simulink model "LogicalArchitecture"  (R2020b)
settings: Solver=VariableStepAuto  StartTime=0.0  StopTime=10.0  RelTol=1e-3
settings Model: DataDictionary=SignalInterfacesDD.sldd  OrderedModelArguments=off  Creator=jantonio  LastModifiedBy=jantonio

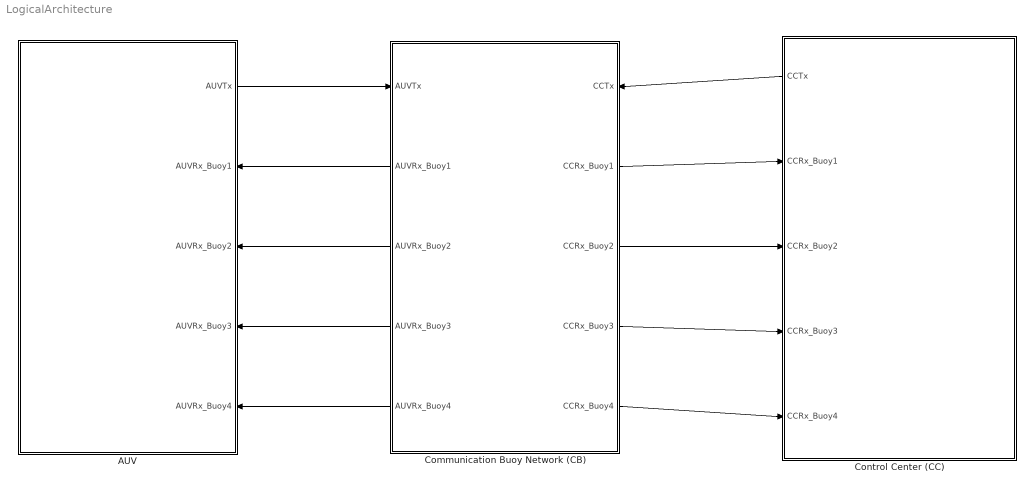
== system LogicalArchitecture ==
  AUV : Subsystem
      settings: PortSchema="{\"entries\":[{\"content\":{\"headerSize\":26,\"margin\":15,\"minimumSpacing\":25,\"sides\":[{\"content\":{\"connectorIds\":[]},\"type\":\"ConnectorPlacement.EquallySpacedRectSide\",\"uuid\":\"7765e1d4-0dc4-4e3a-8ace-6707e97be0d4\"},{\"content\":{\"connectorIds\":[\"Out1\",\"In1\",\"In2\",\"In3\",\"In4\"],\"side\":\"RIGHT\"},\"type\":\"ConnectorPlacement.EquallySpacedRectSide\",\"uuid\":\"17453679-37e1-41d9-ae4d-157eecb5c7d5\"},{\"content\":{\"connectorIds\":[],\"side\":\"TOP\"},\"type\":\"ConnectorPlacement.EquallySpacedRectSide\",\"uuid\":\"00031b71-5a14-4188-ab65-fea9bc3c8fe0\"},{\"content\":{\"connectorIds\":[],\"side\":\"HIDDEN\"},\"type\":\"ConnectorPlacement.EquallySpacedRectSide\",\"uuid\":\"5a9649b7-70c5-4a2b-8171-d74ca0553427\"}]},\"type\":\"ConnectorPlacement.EquallySpacedConnector\",\"uuid\":\"792023c5-1206-4f5a-b9db-8c0c10ca5715\"}],\"packageUris\":[\"http://schema.mathworks.com/mf0/Connector/R2020b\"],\"version\":\"1.0\"}"
  Communication Buoy Network (CB) : Subsystem
      settings: PortSchema="{\"entries\":[{\"content\":{\"headerSize\":26,\"margin\":15,\"minimumSpacing\":25,\"sides\":[{\"content\":{\"connectorIds\":[\"In1\",\"Out5\",\"Out8\",\"Out7\",\"Out6\"]},\"type\":\"ConnectorPlacement.EquallySpacedRectSide\",\"uuid\":\"7765e1d4-0dc4-4e3a-8ace-6707e97be0d4\"},{\"content\":{\"connectorIds\":[\"In2\",\"Out1\",\"Out2\",\"Out3\",\"Out4\"],\"side\":\"RIGHT\"},\"type\":\"ConnectorPlacement.EquallySpacedRectSide\",\"uuid\":\"17453679-37e1-41d9-ae4d-157eecb5c7d5\"},{\"content\":{\"connectorIds\":[],\"side\":\"TOP\"},\"type\":\"ConnectorPlacement.EquallySpacedRectSide\",\"uuid\":\"00031b71-5a14-4188-ab65-fea9bc3c8fe0\"},{\"content\":{\"connectorIds\":[],\"side\":\"HIDDEN\"},\"type\":\"ConnectorPlacement.EquallySpacedRectSide\",\"uuid\":\"5a9649b7-70c5-4a2b-8171-d74ca0553427\"}]},\"type\":\"ConnectorPlacement.EquallySpacedConnector\",\"uuid\":\"792023c5-1206-4f5a-b9db-8c0c10ca5715\"}],\"packageUris\":[\"http://schema.mathworks.com/mf0/Connector/R2020b\"],\"version\":\"1.0\"}"
  Control Center (CC) : Subsystem
      settings: PortSchema="{\"entries\":[{\"content\":{\"headerSize\":26,\"margin\":15,\"minimumSpacing\":25,\"sides\":[{\"content\":{\"connectorIds\":[\"Out1\",\"In1\",\"In2\",\"In3\",\"In4\"]},\"type\":\"ConnectorPlacement.EquallySpacedRectSide\",\"uuid\":\"5928ce2f-b7da-4eaf-83b8-f1dfd8275719\"},{\"content\":{\"connectorIds\":[],\"side\":\"RIGHT\"},\"type\":\"ConnectorPlacement.EquallySpacedRectSide\",\"uuid\":\"1e52cfd1-9d99-4f69-bb2a-b495e37ce87e\"},{\"content\":{\"connectorIds\":[],\"side\":\"TOP\"},\"type\":\"ConnectorPlacement.EquallySpacedRectSide\",\"uuid\":\"b4ddd4ca-36f1-4266-858a-a649bf629535\"},{\"content\":{\"connectorIds\":[],\"side\":\"HIDDEN\"},\"type\":\"ConnectorPlacement.EquallySpacedRectSide\",\"uuid\":\"84c51e85-8df3-4dbb-bd65-3b1aecd54e94\"}]},\"type\":\"ConnectorPlacement.EquallySpacedConnector\",\"uuid\":\"e0d55cd3-5fe9-4d4e-95d9-79589f5b6259\"}],\"packageUris\":[\"http://schema.mathworks.com/mf0/Connector/R2020b\"],\"version\":\"1.0\"}"
  wires:
  AUV/1(AUVTx) -> Communication Buoy Network (CB)/1(AUVTx)
  Control Center (CC)/1(CCTx) -> Communication Buoy Network (CB)/2(CCTx)
  Communication Buoy Network (CB)/5(AUVRx_Buoy1) -> AUV/1(AUVRx_Buoy1)
  Communication Buoy Network (CB)/8(AUVRx_Buoy2) -> AUV/2(AUVRx_Buoy2)
  Communication Buoy Network (CB)/7(AUVRx_Buoy3) -> AUV/3(AUVRx_Buoy3)
  Communication Buoy Network (CB)/6(AUVRx_Buoy4) -> AUV/4(AUVRx_Buoy4)
  Communication Buoy Network (CB)/1(CCRx_Buoy1) -> Control Center (CC)/1(CCRx_Buoy1)
  Communication Buoy Network (CB)/2(CCRx_Buoy2) -> Control Center (CC)/2(CCRx_Buoy2)
  Communication Buoy Network (CB)/3(CCRx_Buoy3) -> Control Center (CC)/3(CCRx_Buoy3)
  Communication Buoy Network (CB)/4(CCRx_Buoy4) -> Control Center (CC)/4(CCRx_Buoy4)

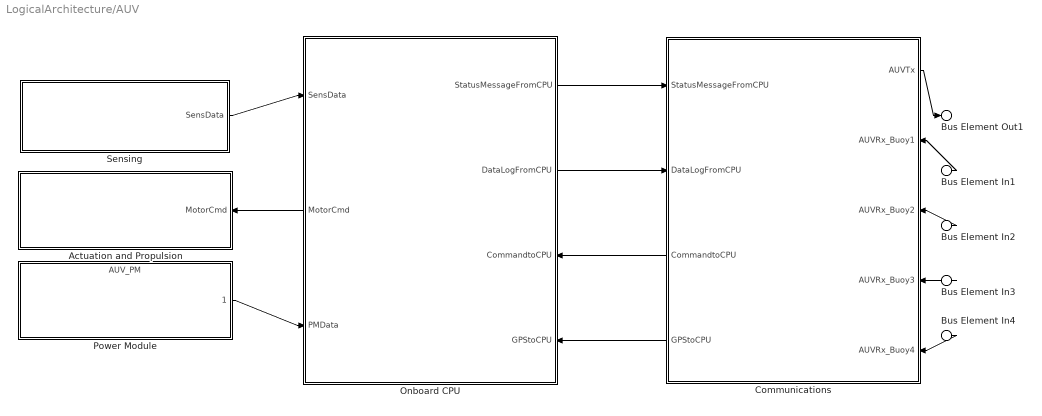
== system LogicalArchitecture/AUV ==
  Bus Element In1 : Inport  PortName=AUVRx_Buoy1
  Bus Element In2 : Inport  Port=2  PortName=AUVRx_Buoy2
  Bus Element In3 : Inport  Port=3  PortName=AUVRx_Buoy3
  Bus Element In4 : Inport  Port=4  PortName=AUVRx_Buoy4
  Actuation and Propulsion : Subsystem
      settings: PortSchema="{\"entries\":[{\"content\":{\"headerSize\":26,\"margin\":15,\"minimumSpacing\":25,\"sides\":[{\"content\":{\"connectorIds\":[]},\"type\":\"ConnectorPlacement.EquallySpacedRectSide\",\"uuid\":\"7765e1d4-0dc4-4e3a-8ace-6707e97be0d4\"},{\"content\":{\"connectorIds\":[\"In1\"],\"side\":\"RIGHT\"},\"type\":\"ConnectorPlacement.EquallySpacedRectSide\",\"uuid\":\"17453679-37e1-41d9-ae4d-157eecb5c7d5\"},{\"content\":{\"connectorIds\":[],\"side\":\"TOP\"},\"type\":\"ConnectorPlacement.EquallySpacedRectSide\",\"uuid\":\"00031b71-5a14-4188-ab65-fea9bc3c8fe0\"},{\"content\":{\"connectorIds\":[],\"side\":\"HIDDEN\"},\"type\":\"ConnectorPlacement.EquallySpacedRectSide\",\"uuid\":\"5a9649b7-70c5-4a2b-8171-d74ca0553427\"}]},\"type\":\"ConnectorPlacement.EquallySpacedConnector\",\"uuid\":\"792023c5-1206-4f5a-b9db-8c0c10ca5715\"}],\"packageUris\":[\"http://schema.mathworks.com/mf0/Connector/R2020b\"],\"version\":\"1.0\"}"
  Communications : Subsystem
      settings: PortSchema="{\"entries\":[{\"content\":{\"headerSize\":26,\"margin\":15,\"minimumSpacing\":25,\"sides\":[{\"content\":{\"connectorIds\":[\"In1\",\"In2\",\"Out2\",\"Out3\"]},\"type\":\"ConnectorPlacement.EquallySpacedRectSide\",\"uuid\":\"5928ce2f-b7da-4eaf-83b8-f1dfd8275719\"},{\"content\":{\"connectorIds\":[\"Out1\",\"In3\",\"In6\",\"In5\",\"In4\"],\"side\":\"RIGHT\"},\"type\":\"ConnectorPlacement.EquallySpacedRectSide\",\"uuid\":\"1e52cfd1-9d99-4f69-bb2a-b495e37ce87e\"},{\"content\":{\"connectorIds\":[],\"side\":\"TOP\"},\"type\":\"ConnectorPlacement.EquallySpacedRectSide\",\"uuid\":\"b4ddd4ca-36f1-4266-858a-a649bf629535\"},{\"content\":{\"connectorIds\":[],\"side\":\"HIDDEN\"},\"type\":\"ConnectorPlacement.EquallySpacedRectSide\",\"uuid\":\"84c51e85-8df3-4dbb-bd65-3b1aecd54e94\"}]},\"type\":\"ConnectorPlacement.EquallySpacedConnector\",\"uuid\":\"e0d55cd3-5fe9-4d4e-95d9-79589f5b6259\"}],\"packageUris\":[\"http://schema.mathworks.com/mf0/Connector/R2020b\"],\"version\":\"1.0\"}"
  Onboard CPU : Subsystem
      settings: PortSchema="{\"entries\":[{\"content\":{\"headerSize\":26,\"margin\":15,\"minimumSpacing\":25,\"sides\":[{\"content\":{\"connectorIds\":[\"In3\",\"Out1\",\"In4\"]},\"type\":\"ConnectorPlacement.EquallySpacedRectSide\",\"uuid\":\"7765e1d4-0dc4-4e3a-8ace-6707e97be0d4\"},{\"content\":{\"connectorIds\":[\"Out3\",\"Out2\",\"In1\",\"In2\"],\"side\":\"RIGHT\"},\"type\":\"ConnectorPlacement.EquallySpacedRectSide\",\"uuid\":\"17453679-37e1-41d9-ae4d-157eecb5c7d5\"},{\"content\":{\"connectorIds\":[],\"side\":\"TOP\"},\"type\":\"ConnectorPlacement.EquallySpacedRectSide\",\"uuid\":\"00031b71-5a14-4188-ab65-fea9bc3c8fe0\"},{\"content\":{\"connectorIds\":[],\"side\":\"HIDDEN\"},\"type\":\"ConnectorPlacement.EquallySpacedRectSide\",\"uuid\":\"5a9649b7-70c5-4a2b-8171-d74ca0553427\"}]},\"type\":\"ConnectorPlacement.EquallySpacedConnector\",\"uuid\":\"792023c5-1206-4f5a-b9db-8c0c10ca5715\"}],\"packageUris\":[\"http://schema.mathworks.com/mf0/Connector/R2020b\"],\"version\":\"1.0\"}"
  Power Module : ModelReference  ModelNameDialog=AUV_PM  SimulationMode=Normal  ModelReferenceVersion=1.7
      settings: PortSchema="{\"entries\":[{\"content\":{\"headerSize\":38,\"margin\":15,\"minimumSpacing\":25,\"sides\":[{\"content\":{\"connectorIds\":[]},\"type\":\"ConnectorPlacement.EquallySpacedRectSide\",\"uuid\":\"7765e1d4-0dc4-4e3a-8ace-6707e97be0d4\"},{\"content\":{\"connectorIds\":[\"Out1\"],\"side\":\"RIGHT\"},\"type\":\"ConnectorPlacement.EquallySpacedRectSide\",\"uuid\":\"17453679-37e1-41d9-ae4d-157eecb5c7d5\"},{\"content\":{\"connectorIds\":[],\"side\":\"TOP\"},\"type\":\"ConnectorPlacement.EquallySpacedRectSide\",\"uuid\":\"00031b71-5a14-4188-ab65-fea9bc3c8fe0\"},{\"content\":{\"connectorIds\":[],\"side\":\"HIDDEN\"},\"type\":\"ConnectorPlacement.EquallySpacedRectSide\",\"uuid\":\"5a9649b7-70c5-4a2b-8171-d74ca0553427\"}]},\"type\":\"ConnectorPlacement.EquallySpacedConnector\",\"uuid\":\"792023c5-1206-4f5a-b9db-8c0c10ca5715\"}],\"packageUris\":[\"http://schema.mathworks.com/mf0/Connector/R2020b\"],\"version\":\"1.0\"}"
  Sensing : Subsystem
      settings: PortSchema="{\"entries\":[{\"content\":{\"headerSize\":26,\"margin\":15,\"minimumSpacing\":25,\"sides\":[{\"content\":{\"connectorIds\":[]},\"type\":\"ConnectorPlacement.EquallySpacedRectSide\",\"uuid\":\"7765e1d4-0dc4-4e3a-8ace-6707e97be0d4\"},{\"content\":{\"connectorIds\":[\"Out1\"],\"side\":\"RIGHT\"},\"type\":\"ConnectorPlacement.EquallySpacedRectSide\",\"uuid\":\"17453679-37e1-41d9-ae4d-157eecb5c7d5\"},{\"content\":{\"connectorIds\":[],\"side\":\"TOP\"},\"type\":\"ConnectorPlacement.EquallySpacedRectSide\",\"uuid\":\"00031b71-5a14-4188-ab65-fea9bc3c8fe0\"},{\"content\":{\"connectorIds\":[],\"side\":\"HIDDEN\"},\"type\":\"ConnectorPlacement.EquallySpacedRectSide\",\"uuid\":\"5a9649b7-70c5-4a2b-8171-d74ca0553427\"}]},\"type\":\"ConnectorPlacement.EquallySpacedConnector\",\"uuid\":\"792023c5-1206-4f5a-b9db-8c0c10ca5715\"}],\"packageUris\":[\"http://schema.mathworks.com/mf0/Connector/R2020b\"],\"version\":\"1.0\"}"
  Bus Element Out1 : Outport  PortName=AUVTx
  wires:
  Power Module/1 -> Onboard CPU/4(PMData)
  Sensing/1(SensData) -> Onboard CPU/3(SensData)
  Onboard CPU/1(MotorCmd) -> Actuation and Propulsion/1(MotorCmd)
  Bus Element In1/1 -> Communications/3(AUVRx_Buoy1)
  Bus Element In2/1 -> Communications/6(AUVRx_Buoy2)
  Bus Element In3/1 -> Communications/5(AUVRx_Buoy3)
  Bus Element In4/1 -> Communications/4(AUVRx_Buoy4)
  Onboard CPU/2(DataLogFromCPU) -> Communications/2(DataLogFromCPU)
  Onboard CPU/3(StatusMessageFromCPU) -> Communications/1(StatusMessageFromCPU)
  Communications/1(AUVTx) -> Bus Element Out1/1
  Communications/2(CommandtoCPU) -> Onboard CPU/1(CommandtoCPU)
  Communications/3(GPStoCPU) -> Onboard CPU/2(GPStoCPU)

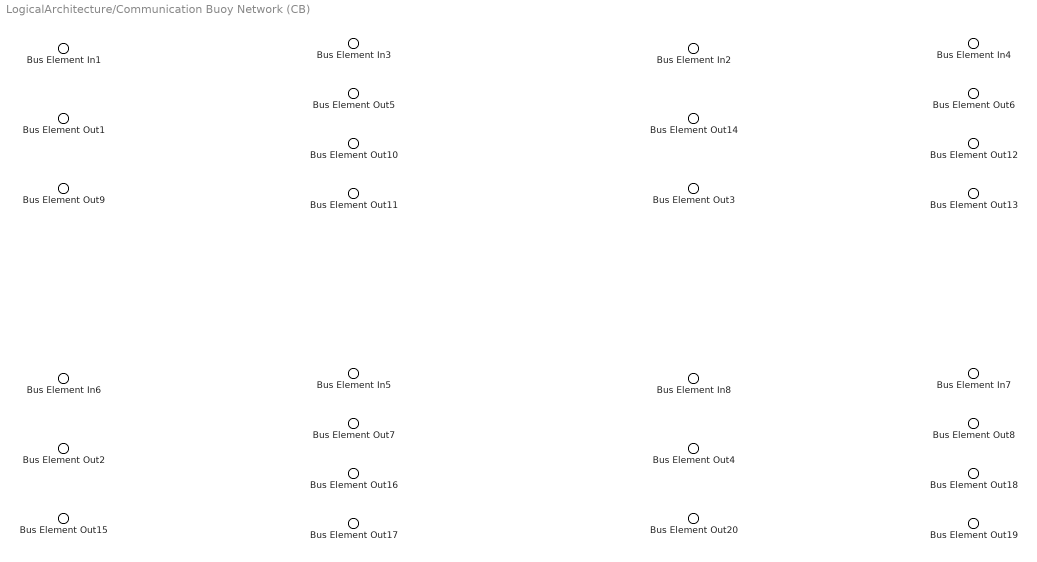
== system LogicalArchitecture/Communication Buoy Network (CB) ==
  Bus Element In{1..2,6,8} (4 alike) : Inport  PortName=AUVTx
  Bus Element In{3..5,7} (4 alike) : Inport  Port=2  PortName=CCTx
  Bus Element Out5 : Outport  PortName=CCRx_Buoy1  Element=StatusMessage
  Bus Element Out10 : Outport  PortName=CCRx_Buoy1  Element=GPS
  Bus Element Out11 : Outport  PortName=CCRx_Buoy1  Element=PowerStatus
  Bus Element Out6 : Outport  Port=2  PortName=CCRx_Buoy2  Element=StatusMessage
  Bus Element Out12 : Outport  Port=2  PortName=CCRx_Buoy2  Element=GPS
  Bus Element Out13 : Outport  Port=2  PortName=CCRx_Buoy2  Element=PowerStatus
  Bus Element Out7 : Outport  Port=3  PortName=CCRx_Buoy3  Element=StatusMessage
  Bus Element Out16 : Outport  Port=3  PortName=CCRx_Buoy3  Element=GPS
  Bus Element Out17 : Outport  Port=3  PortName=CCRx_Buoy3  Element=PowerStatus
  Bus Element Out8 : Outport  Port=4  PortName=CCRx_Buoy4  Element=StatusMessage
  Bus Element Out18 : Outport  Port=4  PortName=CCRx_Buoy4  Element=GPS
  Bus Element Out19 : Outport  Port=4  PortName=CCRx_Buoy4  Element=PowerStatus
  Bus Element Out1 : Outport  Port=5  PortName=AUVRx_Buoy1  Element=GPS
  Bus Element Out9 : Outport  Port=5  PortName=AUVRx_Buoy1  Element=Command
  Bus Element Out4 : Outport  Port=6  PortName=AUVRx_Buoy4  Element=GPS
  Bus Element Out20 : Outport  Port=6  PortName=AUVRx_Buoy4  Element=Command
  Bus Element Out2 : Outport  Port=7  PortName=AUVRx_Buoy3  Element=GPS
  Bus Element Out15 : Outport  Port=7  PortName=AUVRx_Buoy3  Element=Command
  Bus Element Out14 : Outport  Port=8  PortName=AUVRx_Buoy2  Element=GPS
  Bus Element Out3 : Outport  Port=8  PortName=AUVRx_Buoy2  Element=Command

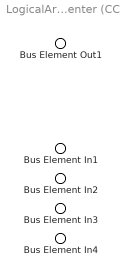
== system LogicalArchitecture/Control Center (CC) ==
  Bus Element In1 : Inport  PortName=CCRx_Buoy1
  Bus Element In2 : Inport  Port=2  PortName=CCRx_Buoy2
  Bus Element In3 : Inport  Port=3  PortName=CCRx_Buoy3
  Bus Element In4 : Inport  Port=4  PortName=CCRx_Buoy4
  Bus Element Out1 : Outport  PortName=CCTx  Element=Command

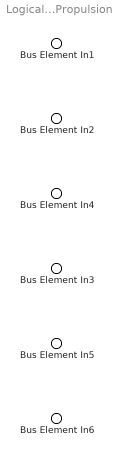
== system LogicalArchitecture/AUV/Actuation and Propulsion ==
  Bus Element In1 : Inport  PortName=MotorCmd  Element=HT1
  Bus Element In2 : Inport  PortName=MotorCmd  Element=HT2
  Bus Element In4 : Inport  PortName=MotorCmd  Element=VT1
  Bus Element In3 : Inport  PortName=MotorCmd  Element=VT2
  Bus Element In5 : Inport  PortName=MotorCmd  Element=MT1
  Bus Element In6 : Inport  PortName=MotorCmd  Element=MT2

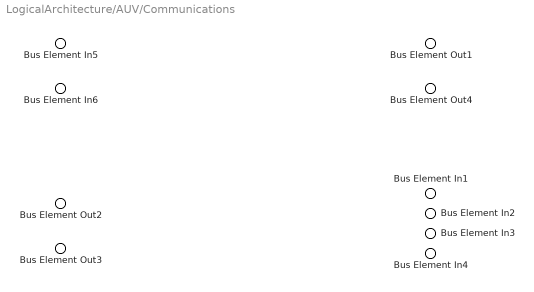
== system LogicalArchitecture/AUV/Communications ==
  Bus Element In5 : Inport  PortName=StatusMessageFromCPU
  Bus Element In6 : Inport  Port=2  PortName=DataLogFromCPU
  Bus Element In1 : Inport  Port=3  PortName=AUVRx_Buoy1
  Bus Element In4 : Inport  Port=4  PortName=AUVRx_Buoy4
  Bus Element In3 : Inport  Port=5  PortName=AUVRx_Buoy3
  Bus Element In2 : Inport  Port=6  PortName=AUVRx_Buoy2
  Bus Element Out1 : Outport  PortName=AUVTx  Element=StatusMessage
  Bus Element Out4 : Outport  PortName=AUVTx  Element=DataLog
  Bus Element Out2 : Outport  Port=2  PortName=CommandtoCPU
  Bus Element Out3 : Outport  Port=3  PortName=GPStoCPU

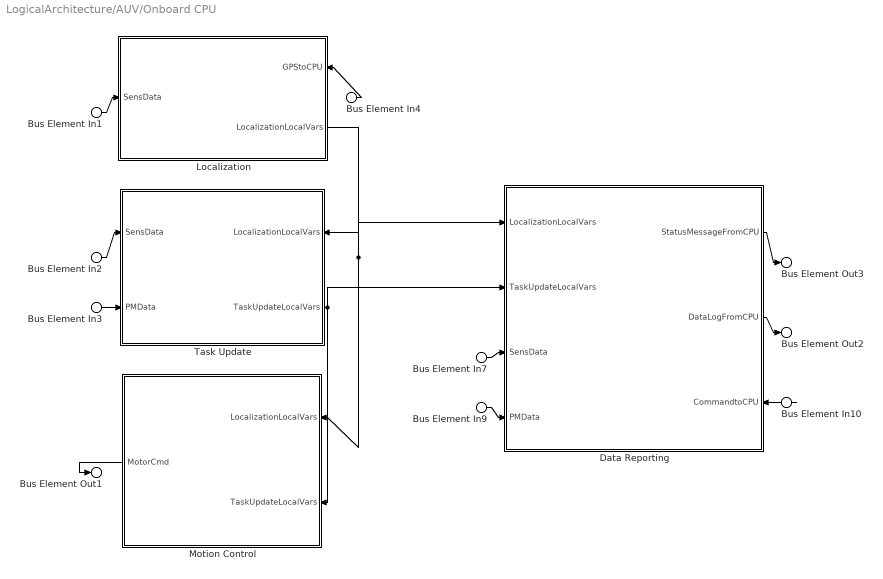
== system LogicalArchitecture/AUV/Onboard CPU ==
  Bus Element In10 : Inport  PortName=CommandtoCPU
  Bus Element In4 : Inport  Port=2  PortName=GPStoCPU
  Bus Element In1 : Inport  Port=3  PortName=SensData
  Bus Element In2 : Inport  Port=3  PortName=SensData
  Bus Element In7 : Inport  Port=3  PortName=SensData
  Bus Element In3 : Inport  Port=4  PortName=PMData
  Bus Element In9 : Inport  Port=4  PortName=PMData
  Data Reporting : Subsystem
      settings: PortSchema="{\"entries\":[{\"content\":{\"headerSize\":26,\"margin\":15,\"minimumSpacing\":25,\"sides\":[{\"content\":{\"connectorIds\":[\"In2\",\"In3\",\"In4\",\"In5\"]},\"type\":\"ConnectorPlacement.EquallySpacedRectSide\",\"uuid\":\"6e074b9a-b44f-4117-a210-2e4c10325222\"},{\"content\":{\"connectorIds\":[\"Out1\",\"Out2\",\"In1\"],\"side\":\"RIGHT\"},\"type\":\"ConnectorPlacement.EquallySpacedRectSide\",\"uuid\":\"4713ac81-953f-4b10-9848-f535a4d44b72\"},{\"content\":{\"connectorIds\":[],\"side\":\"TOP\"},\"type\":\"ConnectorPlacement.EquallySpacedRectSide\",\"uuid\":\"8be01676-2108-4059-a023-470a4c35f4bf\"},{\"content\":{\"connectorIds\":[],\"side\":\"HIDDEN\"},\"type\":\"ConnectorPlacement.EquallySpacedRectSide\",\"uuid\":\"431e50f5-d6e2-4418-bd90-db3bcd3c5653\"}]},\"type\":\"ConnectorPlacement.EquallySpacedConnector\",\"uuid\":\"7eb13a87-3224-4b60-a5bd-7499c6510f09\"}],\"packageUris\":[\"http://schema.mathworks.com/mf0/Connector/R2020b\"],\"version\":\"1.0\"}"
  Localization : Subsystem
      settings: PortSchema="{\"entries\":[{\"content\":{\"headerSize\":26,\"margin\":15,\"minimumSpacing\":25,\"sides\":[{\"content\":{\"connectorIds\":[\"In1\"]},\"type\":\"ConnectorPlacement.EquallySpacedRectSide\",\"uuid\":\"d7fd4b25-d7f9-480e-9c1f-219c1b7124b0\"},{\"content\":{\"connectorIds\":[\"In2\",\"Out1\"],\"side\":\"RIGHT\"},\"type\":\"ConnectorPlacement.EquallySpacedRectSide\",\"uuid\":\"9844324b-a41b-4b87-b09a-567239ca4ffd\"},{\"content\":{\"connectorIds\":[],\"side\":\"TOP\"},\"type\":\"ConnectorPlacement.EquallySpacedRectSide\",\"uuid\":\"bd7c958e-edb2-436c-88f2-21a7aa5ac50b\"},{\"content\":{\"connectorIds\":[],\"side\":\"BOTTOM\"},\"type\":\"ConnectorPlacement.EquallySpacedRectSide\",\"uuid\":\"bfe01049-83d5-4e47-9312-beffa89a52cd\"},{\"content\":{\"connectorIds\":[],\"side\":\"HIDDEN\"},\"type\":\"ConnectorPlacement.EquallySpacedRectSide\",\"uuid\":\"73008776-1040-4b37-a6ad-8079aa15139d\"}]},\"type\":\"ConnectorPlacement.EquallySpacedConnector\",\"uuid\":\"ac73151f-8b38-4e86-8932-e2c7087bb835\"}],\"packageUris\":[\"http://schema.mathworks.com/mf0/Connector/R2020b\"],\"version\":\"1.0\"}"
  Motion Control : Subsystem
      settings: PortSchema="{\"entries\":[{\"content\":{\"headerSize\":26,\"margin\":15,\"minimumSpacing\":25,\"sides\":[{\"content\":{\"connectorIds\":[\"Out1\"]},\"type\":\"ConnectorPlacement.EquallySpacedRectSide\",\"uuid\":\"d7fd4b25-d7f9-480e-9c1f-219c1b7124b0\"},{\"content\":{\"connectorIds\":[\"In2\",\"In1\"],\"side\":\"RIGHT\"},\"type\":\"ConnectorPlacement.EquallySpacedRectSide\",\"uuid\":\"9844324b-a41b-4b87-b09a-567239ca4ffd\"},{\"content\":{\"connectorIds\":[],\"side\":\"TOP\"},\"type\":\"ConnectorPlacement.EquallySpacedRectSide\",\"uuid\":\"bd7c958e-edb2-436c-88f2-21a7aa5ac50b\"},{\"content\":{\"connectorIds\":[],\"side\":\"HIDDEN\"},\"type\":\"ConnectorPlacement.EquallySpacedRectSide\",\"uuid\":\"73008776-1040-4b37-a6ad-8079aa15139d\"}]},\"type\":\"ConnectorPlacement.EquallySpacedConnector\",\"uuid\":\"ac73151f-8b38-4e86-8932-e2c7087bb835\"}],\"packageUris\":[\"http://schema.mathworks.com/mf0/Connector/R2020b\"],\"version\":\"1.0\"}"
  Task Update : Subsystem
      settings: PortSchema="{\"entries\":[{\"content\":{\"headerSize\":26,\"margin\":15,\"minimumSpacing\":25,\"sides\":[{\"content\":{\"connectorIds\":[\"In1\",\"In2\"]},\"type\":\"ConnectorPlacement.EquallySpacedRectSide\",\"uuid\":\"d7fd4b25-d7f9-480e-9c1f-219c1b7124b0\"},{\"content\":{\"connectorIds\":[\"In3\",\"Out1\"],\"side\":\"RIGHT\"},\"type\":\"ConnectorPlacement.EquallySpacedRectSide\",\"uuid\":\"9844324b-a41b-4b87-b09a-567239ca4ffd\"},{\"content\":{\"connectorIds\":[],\"side\":\"TOP\"},\"type\":\"ConnectorPlacement.EquallySpacedRectSide\",\"uuid\":\"bd7c958e-edb2-436c-88f2-21a7aa5ac50b\"},{\"content\":{\"connectorIds\":[],\"side\":\"BOTTOM\"},\"type\":\"ConnectorPlacement.EquallySpacedRectSide\",\"uuid\":\"0ee64a5e-b9ba-437b-ab07-a46302fac79f\"},{\"content\":{\"connectorIds\":[],\"side\":\"HIDDEN\"},\"type\":\"ConnectorPlacement.EquallySpacedRectSide\",\"uuid\":\"73008776-1040-4b37-a6ad-8079aa15139d\"}]},\"type\":\"ConnectorPlacement.EquallySpacedConnector\",\"uuid\":\"ac73151f-8b38-4e86-8932-e2c7087bb835\"}],\"packageUris\":[\"http://schema.mathworks.com/mf0/Connector/R2020b\"],\"version\":\"1.0\"}"
  Bus Element Out1 : Outport  PortName=MotorCmd
  Bus Element Out2 : Outport  Port=2  PortName=DataLogFromCPU
  Bus Element Out3 : Outport  Port=3  PortName=StatusMessageFromCPU
  wires:
  Bus Element In4/1 -> Localization/2(GPStoCPU)
  Bus Element In1/1 -> Localization/1(SensData)
  Localization/1(LocalizationLocalVars) -> Task Update/3(LocalizationLocalVars), Motion Control/2(LocalizationLocalVars), Data Reporting/2(LocalizationLocalVars)
  Bus Element In3/1 -> Task Update/2(PMData)
  Bus Element In2/1 -> Task Update/1(SensData)
  Task Update/1(TaskUpdateLocalVars) -> Motion Control/1(TaskUpdateLocalVars), Data Reporting/3(TaskUpdateLocalVars)
  Motion Control/1(MotorCmd) -> Bus Element Out1/1
  Bus Element In7/1 -> Data Reporting/4(SensData)
  Bus Element In9/1 -> Data Reporting/5(PMData)
  Bus Element In10/1 -> Data Reporting/1(CommandtoCPU)
  Data Reporting/1(StatusMessageFromCPU) -> Bus Element Out3/1
  Data Reporting/2(DataLogFromCPU) -> Bus Element Out2/1

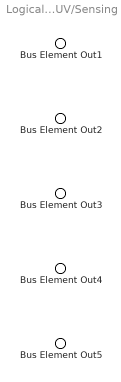
== system LogicalArchitecture/AUV/Sensing ==
  Bus Element Out1 : Outport  PortName=SensData  Element=IMU
  Bus Element Out2 : Outport  PortName=SensData  Element=DVL
  Bus Element Out3 : Outport  PortName=SensData  Element=FoSo
  Bus Element Out4 : Outport  PortName=SensData  Element=DoSo
  Bus Element Out5 : Outport  PortName=SensData  Element=PaSo

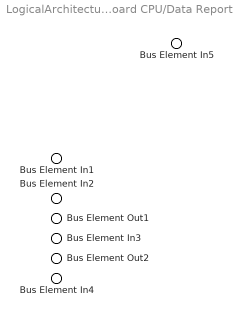
== system LogicalArchitecture/AUV/Onboard CPU/Data Reporting ==
  Bus Element In5 : Inport  PortName=CommandtoCPU
  Bus Element In1 : Inport  Port=2  PortName=LocalizationLocalVars
  Bus Element In2 : Inport  Port=3  PortName=TaskUpdateLocalVars
  Bus Element In3 : Inport  Port=4  PortName=SensData
  Bus Element In4 : Inport  Port=5  PortName=PMData
  Bus Element Out1 : Outport  PortName=StatusMessageFromCPU
  Bus Element Out2 : Outport  Port=2  PortName=DataLogFromCPU

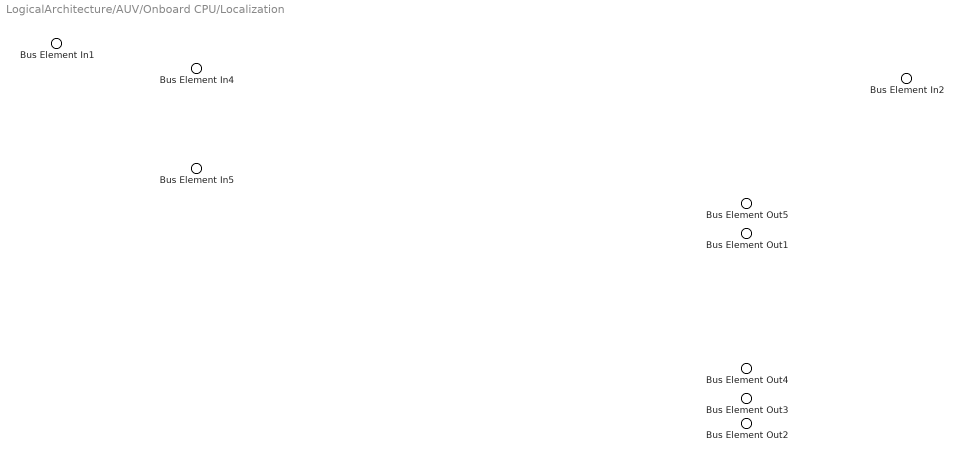
== system LogicalArchitecture/AUV/Onboard CPU/Localization ==
  Bus Element In1 : Inport  PortName=SensData  Element=IMU
  Bus Element In4 : Inport  PortName=SensData  Element=DVL
  Bus Element In5 : Inport  PortName=SensData  Element=DoSo
  Bus Element In2 : Inport  Port=2  PortName=GPStoCPU
  Bus Element Out2 : Outport  PortName=LocalizationLocalVars  Element=SpeedVector
  Bus Element Out3 : Outport  PortName=LocalizationLocalVars  Element=Depth
  Bus Element Out4 : Outport  PortName=LocalizationLocalVars  Element=Pose
  Bus Element Out5 : Outport  PortName=LocalizationLocalVars  Element=GPSLocation
  Bus Element Out1 : Outport  PortName=LocalizationLocalVars  Element=FusedLocation

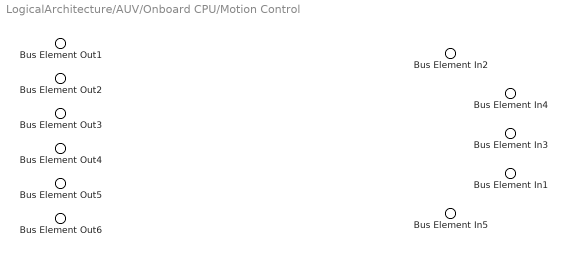
== system LogicalArchitecture/AUV/Onboard CPU/Motion Control ==
  Bus Element In5 : Inport  PortName=TaskUpdateLocalVars  Element=ObstacleVector
  Bus Element In2 : Inport  PortName=TaskUpdateLocalVars  Element=ReferencePath
  Bus Element In1 : Inport  Port=2  PortName=LocalizationLocalVars  Element=SpeedVector
  Bus Element In3 : Inport  Port=2  PortName=LocalizationLocalVars  Element=Pose
  Bus Element In4 : Inport  Port=2  PortName=LocalizationLocalVars  Element=FusedLocation
  Bus Element Out1 : Outport  PortName=MotorCmd  Element=HT1
  Bus Element Out2 : Outport  PortName=MotorCmd  Element=HT2
  Bus Element Out5 : Outport  PortName=MotorCmd  Element=VT1
  Bus Element Out6 : Outport  PortName=MotorCmd  Element=VT2
  Bus Element Out3 : Outport  PortName=MotorCmd  Element=MT1
  Bus Element Out4 : Outport  PortName=MotorCmd  Element=MT2

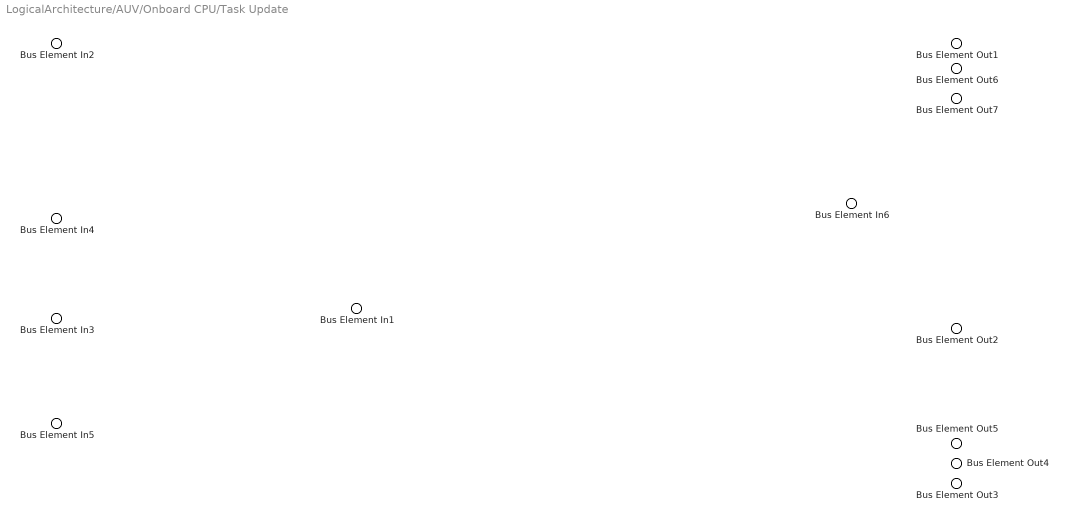
== system LogicalArchitecture/AUV/Onboard CPU/Task Update ==
  Bus Element In2 : Inport  PortName=SensData  Element=FoSo
  Bus Element In5 : Inport  PortName=SensData  Element=DoSo
  Bus Element In4 : Inport  PortName=SensData  Element=PaSo
  Bus Element In3 : Inport  Port=2  PortName=PMData
  Bus Element In6 : Inport  Port=3  PortName=LocalizationLocalVars  Element=FusedLocation
  Bus Element In1 : Inport  Port=3  PortName=LocalizationLocalVars  Element=FusedLocation
  Bus Element Out1 : Outport  PortName=TaskUpdateLocalVars  Element=ObstacleVector
  Bus Element Out7 : Outport  PortName=TaskUpdateLocalVars  Element=TargetStatus
  Bus Element Out6 : Outport  PortName=TaskUpdateLocalVars  Element=TargetLocation
  Bus Element Out5 : Outport  PortName=TaskUpdateLocalVars  Element=SearchParameter
  Bus Element Out2 : Outport  PortName=TaskUpdateLocalVars  Element=ReferencePath
  Bus Element Out4 : Outport  PortName=TaskUpdateLocalVars  Element=MappingParameters
  Bus Element Out3 : Outport  PortName=TaskUpdateLocalVars  Element=MappingData
